simulink model "untitled1"  (R2020a)
settings: Solver=VariableStepAuto  StartTime=0.0  StopTime=10.0  RelTol=1e-3
libraries: lib5 x2
settings Model: Creator=hussein  LastModifiedBy=hussein

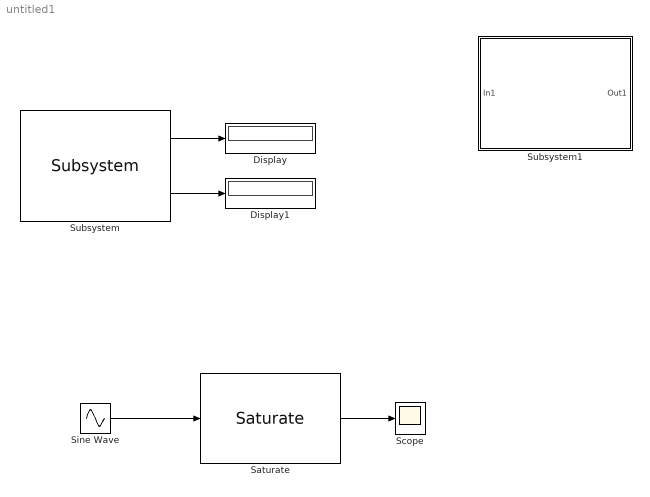
== system untitled1 ==
  Display : Display
  Display1 : Display
  Saturate : lib5/Saturate  U_lim=0.5  L_lim=-0.5
  Scope : Scope
  Sine Wave : Sin  SampleTime=0
  Subsystem : lib5/Subsystem  GAIN=8
  Subsystem1 : Subsystem  AncestorBlock=lib5/Subsystem
      mask Help: abc
      mask Display:
      | disp('My_Block');
      | port_label('input',1,'signal');
      | port_label('output',1,'out');
  wires:
  Subsystem/1 -> Display/1
  Subsystem/2 -> Display1/1
  Sine Wave/1 -> Saturate/1
  Saturate/1 -> Scope/1

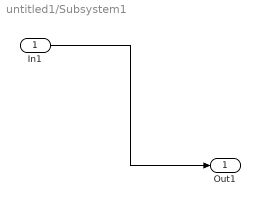
== system untitled1/Subsystem1 ==
  In1 : Inport
  Out1 : Outport
  wires:
  In1/1 -> Out1/1
